simulink model "Verification"  (R2024a)
settings: Solver=FixedStepDiscrete  StartTime=0.0  StopTime=10.0  FixedStep=0.1  RelTol=1e-3
values from neighbouring files (symbols this model uses):
  MIN_SEP_KM = 0.5    [project_params.sldd]
  T_MAX = 100.0    [project_params.sldd]
settings Model: DataDictionary=project_params.sldd  Creator=amir  LastModifiedBy=amir

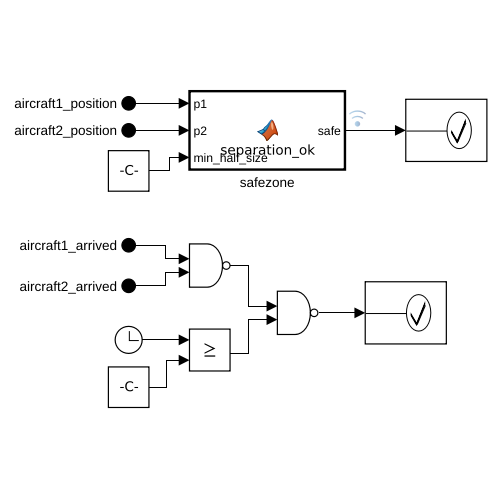
[thumbnail: Simulink's stored preview of the top-level diagram]
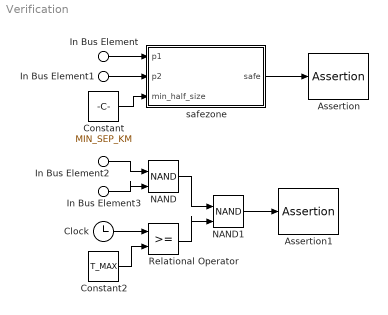
== system Verification ==
  In Bus Element : Inport  PortName=aircraft1_position
  In Bus Element1 : Inport  Port=2  PortName=aircraft2_position
  In Bus Element2 : Inport  Port=3  PortName=aircraft1_arrived
  In Bus Element3 : Inport  Port=4  PortName=aircraft2_arrived
  Assertion : Assertion
  Assertion1 : Assertion
  Clock : Clock
      settings: Decimation=200
  Constant : Constant  Value=MIN_SEP_KM
  Constant2 : Constant  Value=T_MAX
  NAND : Logic  Operator=NAND  IconShape=distinctive  AllPortsSameDT=off  OutDataTypeStr=boolean
  NAND1 : Logic  Operator=NAND  IconShape=distinctive  AllPortsSameDT=off  OutDataTypeStr=boolean
  Relational Operator : RelationalOperator  OutDataTypeStr=boolean  RndMeth=Simplest  InputSameDT=off
  safezone : MATLAB Function  TreatAsAtomicUnit=on
  wires:
  In Bus Element/1 -> safezone/1(p1)
  In Bus Element1/1 -> safezone/2(p2)
  In Bus Element2/1 -> NAND/1
  In Bus Element3/1 -> NAND/2
  Constant/1 -> safezone/3(min_half_size)
  safezone/1(safe) -> Assertion/1
  Clock/1 -> Relational Operator/1
  Constant2/1 -> Relational Operator/2
  NAND/1 -> NAND1/1
  Relational Operator/1 -> NAND1/2
  NAND1/1 -> Assertion1/1

== matlab function Verification/safezone ==
  data: p1 input size=[1, 2]; safe output boolean; p2 input size=[1, 2]; min_half_size input
function safe = separation_ok(p1, p2, min_half_size)
%#codegen
% p1, p2 = [x,y] coordinates (1x2)
dx = abs(round(p1(1) - p2(1)));
dy = abs(round(p1(2) - p2(2)));

% Safe if not BOTH within the danger half-size
safe = ~(dx < min_half_size && dy < min_half_size);
end
